simulink model "BikeWithServo"  (R2018a)
settings: Solver=VariableStepAuto  StartTime=0.0  StopTime=60  RelTol=1e-3
settings Model: Creator=Philip  LastModifiedBy=Philip

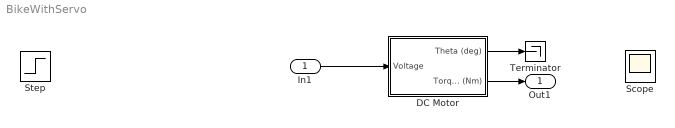
== system BikeWithServo ==
  In1 : Inport
  DC Motor : Subsystem
  Scope : Scope
  Step : Step  Time=10  After=10  SampleTime=0
  Terminator : Terminator
  Out1 : Outport
  wires:
  DC Motor/1(Theta (deg)) -> Terminator/1
  DC Motor/2(Torque (Nm)) -> Out1/1
  In1/1 -> DC Motor/1(Voltage)

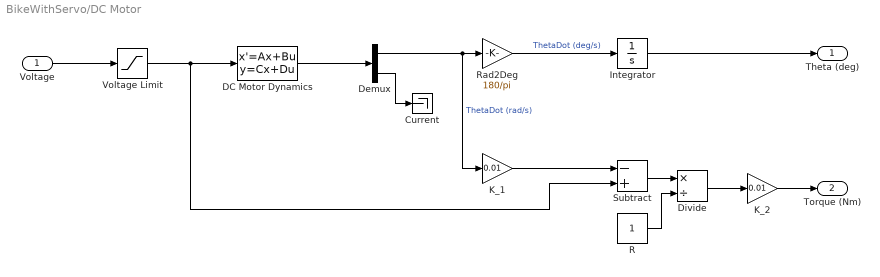
== system BikeWithServo/DC Motor ==
  Voltage : Inport
  Current : Terminator
  DC Motor Dynamics : StateSpace  A=[-10, 1; -0.02, -2]  B=[0; 2]  C=eye(2)  D=zeros(2,1)  InitialCondition=0
  Demux : Demux  Outputs=2
  Divide : Product  Inputs=*/
  Integrator : Integrator
  K_1 : Gain  Gain=0.01
  K_2 : Gain  Gain=0.01
  R : Constant
  Rad2Deg : Gain  Gain=180/pi
  Subtract : Sum  Inputs=-+
  Voltage Limit : Saturate  UpperLimit=12  LowerLimit=0
  Theta (deg) : Outport
  Torque (Nm) : Outport  Port=2
  wires:
  Voltage/1 -> Voltage Limit/1
  Voltage Limit/1 -> Subtract/2, DC Motor Dynamics/1
  DC Motor Dynamics/1 -> Demux/1
  Demux/1 -> K_1/1, Rad2Deg/1  "ThetaDot (rad/s)"
  Rad2Deg/1 -> Integrator/1  "ThetaDot (deg/s)"
  Integrator/1 -> Theta (deg)/1
  Divide/1 -> K_2/1
  K_1/1 -> Subtract/1
  Subtract/1 -> Divide/1
  R/1 -> Divide/2
  K_2/1 -> Torque (Nm)/1
  Demux/2 -> Current/1
